simulink model "Phase_Estimator_1"  (R2020b)
settings: Solver=ode3  StartTime=0.0  StopTime=t(end)  FixedStep=1/60  RelTol=1e-3  EnableMultiTasking=on
undefined symbols (not defined in the file or in its folder): Activity, gamma_d, gamma_omg, x_initial, zeta
settings Model: Creator=wangf7  LastModifiedBy=chukw
settings DataIOCC: LimitDataPoints=on  SaveFormat=Array  ReturnWorkspaceOutputs=off
settings OptimizationCC: ExpressionDepthLimit=2147483647  LifeSpan=inf
settings DebuggingCC: UnderspecifiedInitializationDetection=Classic  MergeDetectMultiDrivingBlocksExec=none  SolverPrmCheckMsg=warning  StateNameClashWarn=warning  SFUnexpectedBacktrackingDiag=warning  SFNoUnconditionalDefaultTransitionDiag=warning  SFExecutionAtInitializationDiag=none  ArithmeticOperatorsInVariantConditions=warning
settings HardwareCC: ProdBitPerPointer=32  ProdBitPerSizeT=32  ProdBitPerPtrDiffT=32  ProdLargestAtomicFloat=None  ProdIntDivRoundTo=Undefined  ProdEndianess=Unspecified  ProdWordSize=32  ProdHWDeviceType=32-bit Generic
settings ModelReferenceCC: PropagateSignalLabelsOutOfModel=off
settings SFSimCC: SimUseLocalCustomCode=off  CustomCodeUndefinedFunction=UseInterfaceOnly
settings RTWCC: RTWUseLocalCustomCode=off
settings CodeAppCC: StateflowObjectComments=on
settings GRTTargetCC: TargetLangStandard=C89/C90 (ANSI)
settings ConfigComp: CovMetricSettings=dw  CovSaveCumulativeToWorkspaceVar=on  CovSaveSingleToWorkspaceVar=on  CovExternalEMLEnable=off
settings SimscapeCC: SimscapeNormalizeSystem=off
settings ConfigurationSet: Description=SimMechanics 2G

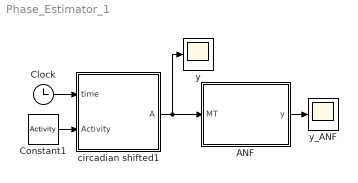
== system Phase_Estimator_1 ==
  ANF : Subsystem
  Clock : Clock
  Constant1 : Constant  Value=Activity
  circadian shifted1 : MATLAB Function  TreatAsAtomicUnit=on
  y : Scope
  y_ANF : Scope
  wires:
  circadian shifted1/1(A) -> y/1, ANF/1(MT)
  Clock/1 -> circadian shifted1/1(time)
  ANF/1(y) -> y_ANF/1
  Constant1/1 -> circadian shifted1/2(Activity)

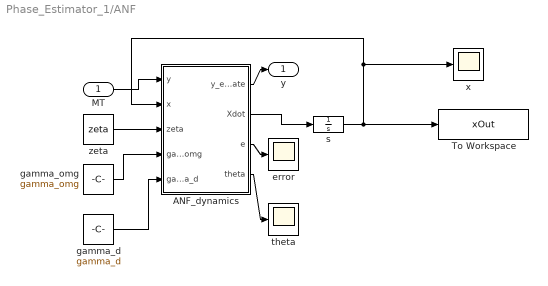
== system Phase_Estimator_1/ANF ==
  MT : Inport
  ANF_dynamics : MATLAB Function  TreatAsAtomicUnit=on
  To Workspace : ToWorkspace  VariableName=xOut  SaveFormat=Timeseries  SampleTime=-1
  error : Scope
  gamma_d : Constant  Value=gamma_d
  gamma_omg : Constant  Value=gamma_omg
  s : Integrator  InitialCondition=x_initial
  theta : Scope
  x : Scope
  zeta : Constant  Value=zeta
  y : Outport
  wires:
  MT/1 -> ANF_dynamics/1(y)
  s/1 -> x/1, ANF_dynamics/2(x), To Workspace/1
  ANF_dynamics/2(Xdot) -> s/1
  ANF_dynamics/1(y_estimate) -> y/1
  ANF_dynamics/3(e) -> error/1
  ANF_dynamics/4(theta) -> theta/1
  zeta/1 -> ANF_dynamics/3(zeta)
  gamma_omg/1 -> ANF_dynamics/4(gamma_omg)
  gamma_d/1 -> ANF_dynamics/5(gamma_d)

== matlab function Phase_Estimator_1/circadian shifted1 ==
  data: time input; Activity input; A output
function A = fcn(time,Activity)
%#eml
A=interp1q(Activity(:,1),Activity(:,2),time);

== matlab function Phase_Estimator_1/ANF/ANF_dynamics ==
  data: y_estimate output; y input; x input; Xdot output; e output; theta output; zeta input; gamma_omg input; gamma_d input
function [y_estimate,Xdot,e,theta] = fcn(y,x,zeta,gamma_omg,gamma_d)

% zeta = 0.03;
% gamma_omg =  0.00000000001;
% gamma_d = 0.0000001;

x1 = x(1);%1st harmonic
x2 = x(2);%1st harmonic dot
dc = x(3);%dc
omg = x(4);%omega

y_estimate = dc + 2*zeta/omg*x2;
e = y - y_estimate;
if isnan(y) || isnan(e)
    e=0;
end

Xdot = zeros(4,1);

Xdot(1,1) = x2;
Xdot(2,1) = omg^2*(e-x1);
Xdot(3,1) = gamma_d*e;
Xdot(4,1) = gamma_omg*(-x1*omg^2)*e;
%y_estimate = dc + 2*zeta/omg*x2;
theta=mod(-atan2(x(2),x(4)*x(1))+pi/2,2*pi);
